simulink model "surgeControl"  (R2015a)
settings: Solver=ode45  StartTime=tstart  StopTime=tstop  RelTol=1e-3
undefined symbols (not defined in the file): c, msfartoystyring, p0, psi0, r0, tsamp, v0
libraries: simulink_extras x3
settings Model: ExtModeAutoUpdateStatusClock=off  Creator=christh  LastModifiedBy=jljoberg
settings DataIOCC: SignalLoggingSaveFormat=ModelDataLogs
settings OptimizationCC: ExpressionDepthLimit=2147483647  InitFltsAndDblsToZero=on
settings DebuggingCC: UnderspecifiedInitializationDetection=Classic  MergeDetectMultiDrivingBlocksExec=none  SolverPrmCheckMsg=warning  StateNameClashWarn=warning
settings GRTTargetCC: CombineOutputUpdateFcns=off  GRTInterface=on
settings ConfigComp: CovMetricSettings=dw  CovHtmlReporting=on  CovSaveCumulativeToWorkspaceVar=on  CovSaveSingleToWorkspaceVar=on  CovExternalEMLEnable=off

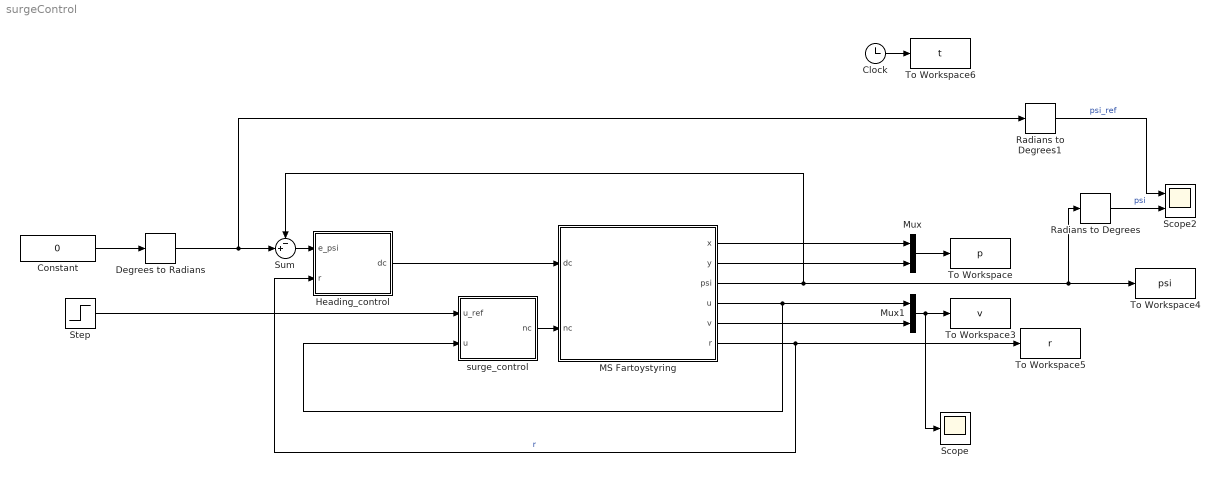
== system surgeControl ==
  Clock : Clock
  Constant : Constant  Value=0
  Degrees to Radians : simulink_extras/Transformations/Degrees to Radians
  Heading_control : Subsystem
  MS Fartoystyring : Subsystem  mask(MS Fartoystyring for Assignment 3 G&C){x0=p0(1), y0=p0(2), u0=v0(1), v0=v0(2), psi0=psi0, r0=r0, c=c}
      mask prompts: x0 "x(t0) (m)"; y0 "y(t0) (m)"; u0 "u(t0) (m/s)"; v0 "v(t0) (m/s)"; psi0 "psi(t0) (rad)"; r0 "r(t0) (rad/s)"; c "current (0 or 1)"
      mask help:
      | Block corresponding to Figure 1 in the assignment text. Gives the response of the ship.
      |
      | The design speed of MS Fartoystyring is u=8.23 m/s.
      |
      | Input:
      | dc: commanded rudder (rad), dmax=25*pi/180
      | nc: commanded shaft speed (rad/s), nmax=85*2*pi/60
      |
      | Output:
      | x: north pos (m)
      | y: east pos (m)
      | u: surge (m/s)
      | v: sway (m/s)
      | psi: heading (rad)
      | r: yaw (rad/s)
      mask Help: Comments, bugs and help requests can be directed to the TA. Email on course website.
  Mux : Mux  Inputs=2
  Mux1 : Mux  Inputs=2
  Radians to Degrees : simulink_extras/Transformations/Radians to Degrees
  Radians to Degrees1 : simulink_extras/Transformations/Radians to Degrees
  Scope : Scope
      settings: YMin=6.98445  YMax=7.01246
  Scope2 : Scope  NumInputPorts=2
      settings: ShowLegends=on  YMin=-0.04402  YMax=0.00489
  Step : Step  Time=500  Before=4  After=7  SampleTime=0
  Sum : Sum  Inputs=-+|
  To Workspace : ToWorkspace  VariableName=p  SampleTime=tsamp
  To Workspace3 : ToWorkspace  VariableName=v  SampleTime=tsamp
  To Workspace4 : ToWorkspace  VariableName=psi  SampleTime=tsamp
  To Workspace5 : ToWorkspace  VariableName=r  SampleTime=tsamp
  To Workspace6 : ToWorkspace  VariableName=t  SampleTime=tsamp
  surge_control : Subsystem
  wires:
  Clock/1 -> To Workspace6/1
  MS Fartoystyring/1(x) -> Mux/1
  MS Fartoystyring/2(y) -> Mux/2
  MS Fartoystyring/4(u) -> surge_control/2(u), Mux1/1
  MS Fartoystyring/5(v) -> Mux1/2
  Mux/1 -> To Workspace/1
  Mux1/1 -> Scope/1, To Workspace3/1
  surge_control/1(nc) -> MS Fartoystyring/2(nc)
  MS Fartoystyring/6(r) -> Heading_control/2(r), To Workspace5/1  "r"
  Sum/1 -> Heading_control/1(e_psi)
  MS Fartoystyring/3(psi) -> Sum/1, Radians to Degrees/1, To Workspace4/1
  Heading_control/1(dc) -> MS Fartoystyring/1(dc)
  Constant/1 -> Degrees to Radians/1
  Radians to Degrees/1 -> Scope2/2  "psi"
  Degrees to Radians/1 -> Sum/2, Radians to Degrees1/1
  Radians to Degrees1/1 -> Scope2/1  "psi_ref"
  Step/1 -> surge_control/1(u_ref)

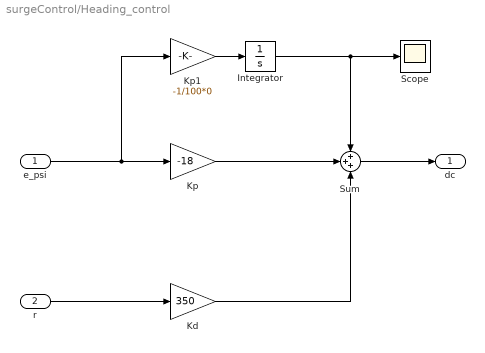
== system surgeControl/Heading_control ==
  e_psi : Inport
  r : Inport  Port=2
  Integrator : Integrator
  Kd : Gain  Gain=350
  Kp : Gain  Gain=-18
  Kp1 : Gain  Gain=-1/100*0
  Scope : Scope
      settings: YMin=-0.01109  YMax=0.01192
  Sum : Sum  Inputs=+++
  dc : Outport
  wires:
  Sum/1 -> dc/1
  e_psi/1 -> Kp1/1, Kp/1
  Kp/1 -> Sum/2
  Kd/1 -> Sum/3
  Kp1/1 -> Integrator/1
  Integrator/1 -> Scope/1, Sum/1
  r/1 -> Kd/1

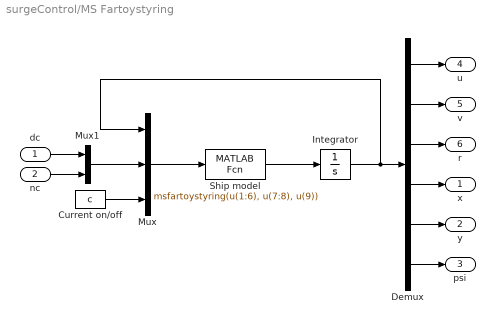
== system surgeControl/MS Fartoystyring ==
  dc : Inport
  nc : Inport  Port=2
  Current on/off : Constant  Value=c
  Demux : Demux  Outputs=6
  Integrator : Integrator  InitialCondition=[u0 v0 r0 x0 y0 psi0]'
  Mux : Mux  Inputs=3
  Mux1 : Mux  Inputs=2
  Ship model : MATLABFcn  MATLABFcn=msfartoystyring(u(1:6), u(7:8), u(9))  OutputDimensions=6
  x : Outport
  y : Outport  Port=2
  psi : Outport  Port=3
  u : Outport  Port=4
  v : Outport  Port=5
  r : Outport  Port=6
  wires:
  Integrator/1 -> Mux/1, Demux/1
  Mux1/1 -> Mux/2
  dc/1 -> Mux1/1
  nc/1 -> Mux1/2
  Demux/1 -> u/1
  Demux/2 -> v/1
  Demux/3 -> r/1
  Demux/4 -> x/1
  Demux/5 -> y/1
  Demux/6 -> psi/1
  Current on/off/1 -> Mux/3
  Ship model/1 -> Integrator/1
  Mux/1 -> Ship model/1

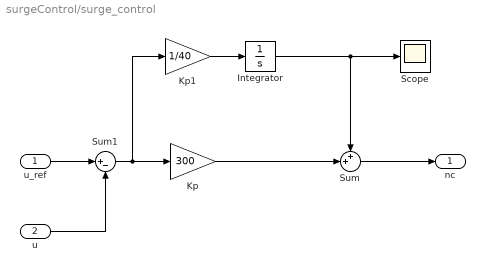
== system surgeControl/surge_control ==
  u_ref : Inport
  u : Inport  Port=2
  Integrator : Integrator  LimitOutput=on  UpperSaturationLimit=8  LowerSaturationLimit=-8
  Kp : Gain  Gain=300
  Kp1 : Gain  Gain=1/40
  Scope : Scope
      settings: YMin=-1.00000  YMax=9.00000
  Sum : Sum  Inputs=++|
  Sum1 : Sum  Inputs=|+-
  nc : Outport
  wires:
  Sum/1 -> nc/1
  Kp/1 -> Sum/2
  Kp1/1 -> Integrator/1
  Integrator/1 -> Scope/1, Sum/1
  u/1 -> Sum1/2
  Sum1/1 -> Kp1/1, Kp/1
  u_ref/1 -> Sum1/1
